simulink model "gm_sampleModel2077_2_sub"  (R2023a)
settings: Solver=VariableStepAuto  StartTime=0.0  StopTime=10.0  RelTol=1e-3
libraries: simulink x1, hdlsllib x1
settings Model: Creator=user1  LastModifiedBy=user1
settings OptimizationCC: BlockReduction=off  ConditionallyExecuteInputs=off
settings DebuggingCC: InheritedTsInSrcMsg=none

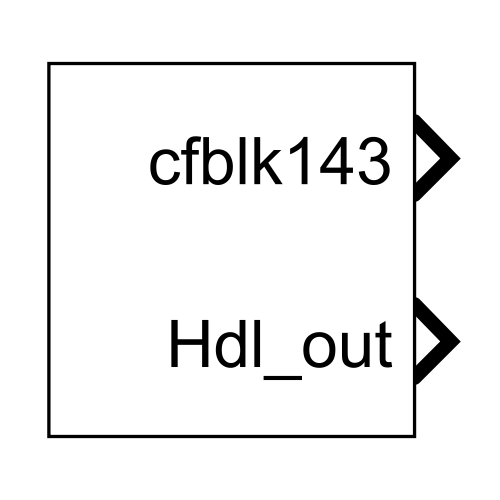
[thumbnail: Simulink's stored preview of the top-level diagram]
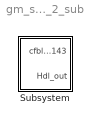
== system gm_sampleModel2077_2_sub ==
  Subsystem : Subsystem

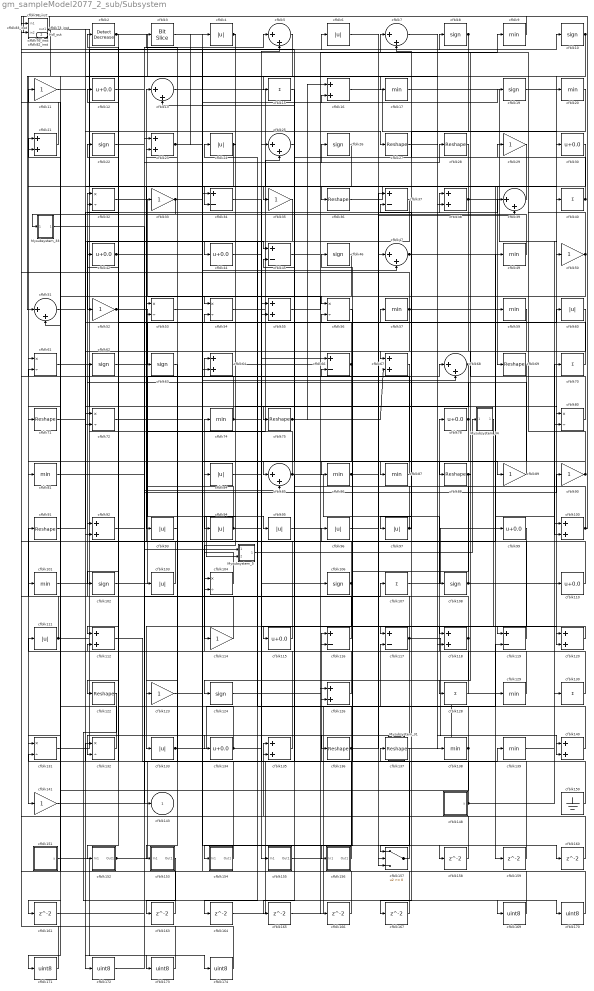
== system gm_sampleModel2077_2_sub/Subsystem ==
  Mysubsystem_31 : Subsystem
  Mysubsystem_33 : Subsystem
  Mysubsystem_34 : Subsystem
  Mysubsystem_5 : Subsystem
  cfblk{8,10,19,22,26,46,62..63,102,106,108,124} (12 alike) : Signum
  cfblk{16,21,23,38,55,64,67,92,100,112,118,120,126,135,140} (15 alike) : Sum  OutDataTypeStr=uint8
  cfblk{9,17,20,49,57,59,74,81,86..87,101,129,138..139} (14 alike) : MinMax  OutDataTypeStr=uint8
  cfblk{4,6,24,60,84,93..97,103,111,133} (13 alike) : Abs  OutDataTypeStr=uint8  SaturateOnIntegerOverflow=off
  cfblk{32,53..54,56,61,72,80,104,131..132} (10 alike) : Product  Inputs=*/  OutDataTypeStr=uint8  RndMeth=Zero  SaturateOnIntegerOverflow=on
  cfblk{15,40,70,107,128,130} (6 alike) : Sum  Inputs=+  OutDataTypeStr=uint8
  cfblk{11,29,33,35,50,52,89..90,114,123,141} (11 alike) : Gain  OutDataTypeStr=uint8
  cfblk{12,30,42,44,78,99,110,115,134} (9 alike) : Bias  Bias=0.0  SaturateOnIntegerOverflow=off
  cfblk{34,37,45,66,116..117,119} (7 alike) : Sum  Inputs=+-  OutDataTypeStr=uint8
  cfblk{27..28,36,69,71,75,88,91,122,136..137} (11 alike) : Reshape
  cfblk127_inst : Subsystem
  cfblk{5,7,13,25,39,47,51,68,85} (9 alike) : Sum  Inputs=|++  OutDataTypeStr=uint8
  cfblk148 : Subsystem  mask(Counter Free-Running){NumBits=double(16), tsamp=double(-1)}
      mask prompts: NumBits "Simulink:masks:NumberOfBits_MP"; tsamp "Simulink:masks:SampleTime_MP"
      mask help: Simulink:masks:CounterFreeRunning_MD
  cfblk14_inst : Subsystem
  cfblk150 : Ground
  cfblk151 : Subsystem  mask(Counter Limited){uplimit=double(7), tsamp=double(-1)}
      mask prompts: uplimit "Simulink:masks:UpperLimit_MP"; tsamp "Simulink:masks:SampleTime_MP"
      mask help: Simulink:masks:CounterLimited_MD
      mask init:
      | nbits = double(8);
      | tsamp = double(-1);
      | uplimit = double(7);
  cfblk152 : Subsystem
  cfblk153 : Subsystem
  cfblk154 : Subsystem
  cfblk155 : Subsystem
  cfblk156 : Subsystem
  cfblk157 : Switch  OutDataTypeStr=uint8  SaturateOnIntegerOverflow=off  InputSameDT=off
  cfblk{158..161,163..167} (9 alike) : Delay  SampleTime=1
  cfblk{169..174} (6 alike) : DataTypeConversion  OutDataTypeStr=uint8  SaturateOnIntegerOverflow=off  RndMeth=Floor
  cfblk18_inst : Subsystem
  cfblk2 : simulink/Logic and Bit Operations/Detect Decrease  vinit=0.0  OutDataTypeStr=uint8
      settings: LibrarySourceBlock=|
      | hdlsllib/Logic and Bit
      | Operations/Detect
      | Decrease
  cfblk3 : hdlsllib/Logic and Bit Operations/Bit Slice  lidx=7  ridx=0
  cfblk58_inst : Subsystem
  cfblk73_inst : Subsystem
  cfblk76_inst : Subsystem
  cfblk82_inst : Subsystem
  cfblk83_inst : Subsystem
  cfblk98_inst : Subsystem
  cfblk143 : Outport  OutDataTypeStr=uint8  SampleTime=1  VectorParamsAs1DForOutWhenUnconnected=off
  Hdl_out : Outport  Port=2  OutDataTypeStr=uint8
  wires:
  Mysubsystem_31/1(Out1) -> cfblk129/1
  Mysubsystem_33/1(Out1) -> Mysubsystem_5/1(In1)
  Mysubsystem_34/1(Out1) -> cfblk117/1
  Mysubsystem_5/1(Out1) -> Mysubsystem_34/1(In1)
  cfblk10/1 -> cfblk120/2, cfblk141/1
  cfblk100/1 -> cfblk14_inst/2(in2), cfblk61/2
  cfblk101/1 -> cfblk6/1
  cfblk102/1 -> cfblk68/1
  cfblk103/1 -> cfblk13/1
  cfblk104/1 -> cfblk74/1
  cfblk106/1 -> cfblk133/1, cfblk32/1
  cfblk107/1 -> cfblk99/1
  cfblk108/1 -> cfblk64/1, cfblk18_inst/1(in1), cfblk110/1
  cfblk11/1 -> cfblk72/1
  cfblk110/1 -> cfblk96/1
  cfblk111/1 -> cfblk91/1, cfblk25/2
  cfblk112/1 -> cfblk135/1
  cfblk114/1 -> cfblk92/1
  cfblk115/1 -> cfblk83_inst/1(in1)
  cfblk116/1 -> cfblk101/1
  cfblk117/1 -> cfblk82_inst/2(in2), cfblk140/2, cfblk127_inst/1(in1), cfblk132/2
  cfblk118/1 -> cfblk83_inst/2(in2), cfblk124/1
  cfblk119/1 -> cfblk11/1
  cfblk12/1 -> cfblk10/1
  cfblk120/1 -> cfblk115/1
  cfblk122/1 -> cfblk170/1
  cfblk123/1 -> cfblk8/1
  cfblk124/1 -> cfblk116/1
  cfblk126/1 -> cfblk84/1
  cfblk127_inst/1(out1) -> cfblk93/1, cfblk69/1, cfblk35/1
  cfblk128/1 -> cfblk78/1
  cfblk129/1 -> cfblk66/2
  cfblk13/1 -> cfblk159/1
  cfblk130/1 -> cfblk111/1
  cfblk131/1 -> cfblk49/1
  cfblk132/1 -> cfblk51/2
  cfblk133/1 -> cfblk119/2, cfblk53/1
  cfblk134/1 -> cfblk25/1, cfblk2/1
  cfblk135/1 -> cfblk24/1
  cfblk136/1 -> cfblk47/1, cfblk116/2, cfblk154/1(In1)
  cfblk137/1 -> cfblk157/1
  cfblk138/1 -> cfblk46/1, cfblk161/1
  cfblk139/1 -> cfblk70/1
  cfblk14_inst/1(out1) -> cfblk45/1, cfblk34/2
  cfblk140/1 -> cfblk54/2
  cfblk141/1 -> cfblk139/1
  cfblk148/1(y) -> cfblk56/2, cfblk132/1, cfblk130/1
  cfblk15/1 -> cfblk85/1
  cfblk150/1 -> cfblk112/2
  cfblk151/1(y) -> cfblk173/1
  cfblk152/1(Out1) -> cfblk55/2, cfblk5/2
  cfblk153/1(Out1) -> cfblk163/1
  cfblk154/1(Out1) -> cfblk23/2
  cfblk155/1(Out1) -> cfblk137/1
  cfblk156/1(Out1) -> cfblk21/1
  cfblk157/1 -> cfblk21/2
  cfblk158/1 -> cfblk58_inst/2(in2)
  cfblk159/1 -> cfblk45/2
  cfblk16/1 -> cfblk30/1
  cfblk160/1 -> cfblk135/2
  cfblk161/1 -> cfblk85/2
  cfblk163/1 -> cfblk23/1
  cfblk164/1 -> cfblk126/2
  cfblk165/1 -> cfblk117/2
  cfblk166/1 -> cfblk131/2
  cfblk167/1 -> cfblk127_inst/2(in2)
  cfblk169/1 -> cfblk34/1
  cfblk17/1 -> cfblk50/1
  cfblk170/1 -> cfblk76_inst/1(in1)
  cfblk171/1 -> cfblk76_inst/2(in2)
  cfblk172/1 -> cfblk107/1
  cfblk173/1 -> cfblk98_inst/1(in1)
  cfblk174/1 -> cfblk98_inst/2(in2)
  cfblk18_inst/1(out1) -> cfblk14_inst/1(in1)
  cfblk19/1 -> cfblk20/1
  cfblk2/1 -> cfblk122/1, cfblk118/2
  cfblk20/1 -> cfblk67/1
  cfblk21/1 -> cfblk82_inst/1(in1)
  cfblk22/1 -> cfblk5/1
  cfblk23/1 -> cfblk95/1, cfblk68/2, cfblk4/1
  cfblk24/1 -> cfblk92/2, cfblk114/1
  cfblk25/1 -> cfblk75/1
  cfblk26/1 -> cfblk71/1
  cfblk27/1 -> cfblk138/1
  cfblk28/1 -> cfblk54/1
  cfblk29/1 -> cfblk61/1
  cfblk3/1 -> cfblk88/1
  cfblk30/1 -> cfblk87/1
  cfblk32/1 -> cfblk166/1
  cfblk33/1 -> cfblk47/2, Mysubsystem_33/1(In1)
  cfblk34/1 -> cfblk155/1(In1)
  cfblk35/1 -> cfblk52/1
  cfblk36/1 -> cfblk40/1
  cfblk37/1 -> cfblk134/1
  cfblk38/1 -> cfblk64/2, cfblk100/1, cfblk33/1
  cfblk39/1 -> cfblk36/1
  cfblk4/1 -> cfblk44/1, cfblk104/2
  cfblk40/1 -> cfblk7/2, cfblk13/2
  cfblk42/1 -> cfblk26/1, cfblk16/2
  cfblk44/1 -> cfblk106/1
  cfblk45/1 -> cfblk9/1
  cfblk46/1 -> cfblk81/1
  cfblk47/1 -> cfblk97/1, cfblk100/2
  cfblk49/1 -> cfblk12/1
  cfblk5/1 -> cfblk131/1
  cfblk50/1 -> cfblk73_inst/2(in2), cfblk112/1
  cfblk51/1 -> cfblk80/1
  cfblk52/1 -> cfblk28/1, Mysubsystem_5/2(In2)
  cfblk53/1 -> cfblk38/1
  cfblk54/1 -> cfblk56/1
  cfblk55/1 -> cfblk19/1
  cfblk56/1 -> cfblk156/1(In1)
  cfblk57/1 -> cfblk18_inst/2(in2), cfblk72/2, cfblk59/1
  cfblk58_inst/1(out1) -> cfblk17/1
  cfblk59/1 -> cfblk128/1
  cfblk6/1 -> cfblk157/2
  cfblk60/1 -> cfblk152/1(In1)
  cfblk61/1 -> cfblk143/1
  cfblk62/1 -> cfblk55/1
  cfblk63/1 -> cfblk153/1(In1)
  cfblk64/1 -> cfblk80/2
  cfblk66/1 -> cfblk42/1, cfblk123/1
  cfblk67/1 -> cfblk94/1
  cfblk68/1 -> cfblk167/1, cfblk104/1
  cfblk69/1 -> cfblk102/1
  cfblk7/1 -> cfblk140/1
  cfblk70/1 -> cfblk32/2
  cfblk71/1 -> cfblk60/1
  cfblk72/1 -> cfblk158/1
  cfblk73_inst/1(out1) -> cfblk27/1
  cfblk74/1 -> cfblk22/1, cfblk89/1
  cfblk75/1 -> cfblk67/2, cfblk16/1
  cfblk76_inst/1(out1) -> cfblk169/1
  cfblk78/1 -> cfblk37/2, cfblk171/1, cfblk164/1
  cfblk8/1 -> cfblk38/2, cfblk15/1
  cfblk80/1 -> cfblk7/1
  cfblk81/1 -> cfblk103/1
  cfblk82_inst/1(out1) -> cfblk174/1
  cfblk83_inst/1(out1) -> cfblk51/1
  cfblk84/1 -> cfblk66/1
  cfblk85/1 -> cfblk108/1, cfblk53/2, cfblk165/1
  cfblk86/1 -> cfblk39/2, cfblk160/1
  cfblk87/1 -> cfblk73_inst/1(in1)
  cfblk88/1 -> cfblk136/1, cfblk118/1
  cfblk89/1 -> cfblk62/1
  cfblk9/1 -> cfblk58_inst/1(in1)
  cfblk90/1 -> cfblk29/1, cfblk86/1
  cfblk91/1 -> cfblk39/1
  cfblk92/1 -> cfblk90/1
  cfblk93/1 -> cfblk3/1
  cfblk94/1 -> cfblk63/1, cfblk120/1
  cfblk95/1 -> cfblk126/1
  cfblk96/1 -> cfblk157/3
  cfblk97/1 -> cfblk37/1, cfblk57/1
  cfblk98_inst/1(out1) -> cfblk172/1
  cfblk99/1 -> cfblk119/1

== system gm_sampleModel2077_2_sub/Subsystem/Mysubsystem_31 ==
  cfblk125_to_const : Constant  Value=double(1)  OutDataTypeStr=double  SampleTime=1
  Out1 : Outport  SampleTime=1
  wires:
  cfblk125_to_const/1 -> Out1/1

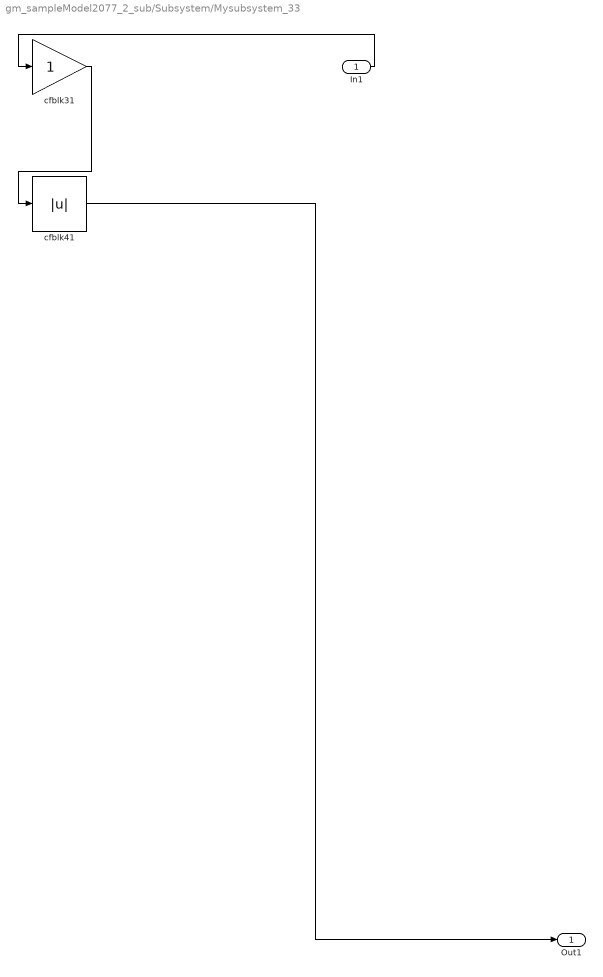
== system gm_sampleModel2077_2_sub/Subsystem/Mysubsystem_33 ==
  In1 : Inport  OutDataTypeStr=uint8  PortDimensions=1  SampleTime=1
  cfblk31 : Gain
  cfblk41 : Abs  SaturateOnIntegerOverflow=off
  Out1 : Outport  SampleTime=1
  wires:
  In1/1 -> cfblk31/1
  cfblk31/1 -> cfblk41/1
  cfblk41/1 -> Out1/1

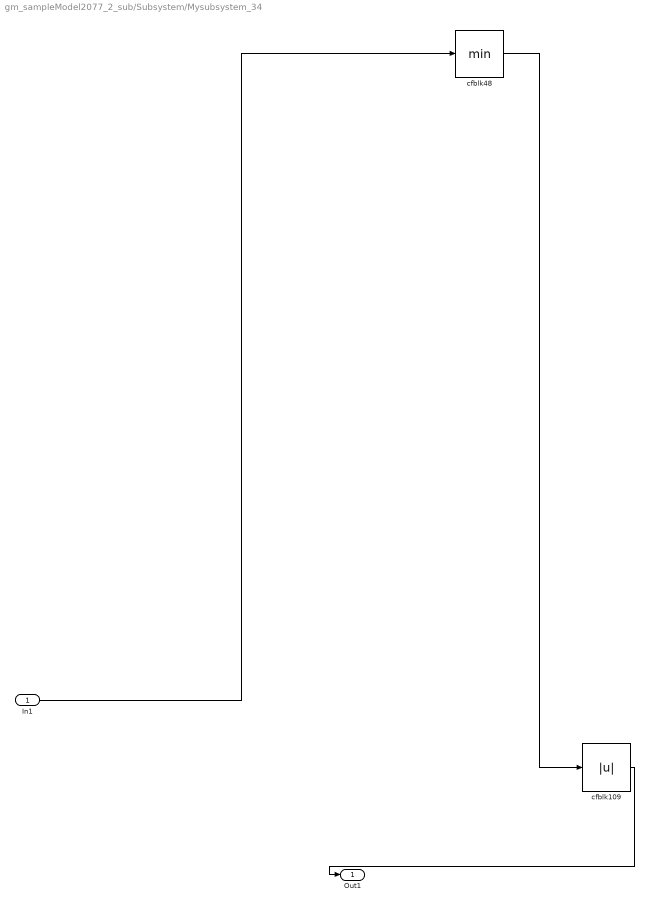
== system gm_sampleModel2077_2_sub/Subsystem/Mysubsystem_34 ==
  In1 : Inport  OutDataTypeStr=fixdt(0, 8, 7)  PortDimensions=1  SampleTime=1
  cfblk109 : Abs  SaturateOnIntegerOverflow=off
  cfblk48 : MinMax
  Out1 : Outport  SampleTime=1
  wires:
  In1/1 -> cfblk48/1
  cfblk109/1 -> Out1/1
  cfblk48/1 -> cfblk109/1

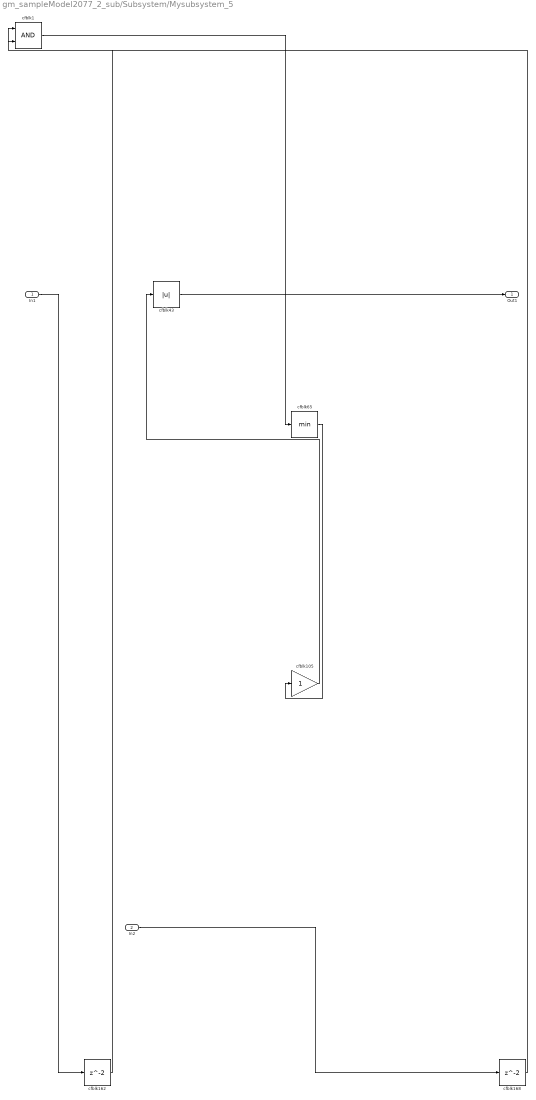
== system gm_sampleModel2077_2_sub/Subsystem/Mysubsystem_5 ==
  In1 : Inport  OutDataTypeStr=fixdt(0, 16, 7)  PortDimensions=1  SampleTime=1
  In2 : Inport  Port=2  OutDataTypeStr=uint8  PortDimensions=1  SampleTime=1
  cfblk1 : Logic  AllPortsSameDT=off  OutDataTypeStr=boolean
  cfblk105 : Gain
  cfblk162 : Delay  SampleTime=1
  cfblk168 : Delay  SampleTime=1
  cfblk43 : Abs  SaturateOnIntegerOverflow=off
  cfblk65 : MinMax
  Out1 : Outport  SampleTime=1
  wires:
  In1/1 -> cfblk162/1
  In2/1 -> cfblk168/1
  cfblk1/1 -> cfblk65/1
  cfblk105/1 -> cfblk43/1
  cfblk162/1 -> cfblk1/1
  cfblk168/1 -> cfblk1/2
  cfblk43/1 -> Out1/1
  cfblk65/1 -> cfblk105/1

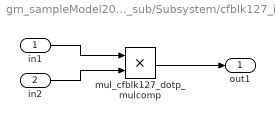
== system gm_sampleModel2077_2_sub/Subsystem/cfblk127_inst ==
  in1 : Inport  OutDataTypeStr=uint8  SampleTime=1
  in2 : Inport  Port=2  OutDataTypeStr=uint8  SampleTime=1
  mul_cfblk127_dotp_mulcomp : Product  Inputs=**  OutDataTypeStr=uint8  SampleTime=1
  out1 : Outport  OutDataTypeStr=uint8  SampleTime=1
  wires:
  in1/1 -> mul_cfblk127_dotp_mulcomp/1
  in2/1 -> mul_cfblk127_dotp_mulcomp/2
  mul_cfblk127_dotp_mulcomp/1 -> out1/1

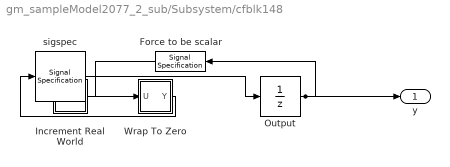
== system gm_sampleModel2077_2_sub/Subsystem/cfblk148 ==
  Force to be scalar : SignalSpecification  DisableCoverage=on  Dimensions=1
  Increment Real World : Subsystem  mask(Real World Value Increment){}
      mask help: Simulink:masks:RealWorldValueIncrement_MD
      mask Display: disp('V++')
  Output : UnitDelay  InitialCondition=0.0  SampleTime=tsamp  HasFrameUpgradeWarning=on
  Wrap To Zero : Subsystem  mask(Wrap To Zero){Threshold=double(65535)}
      mask prompts: Threshold "Simulink:masks:Threshold_MP"
      mask help: Simulink:masks:WrapToZero_MD
  sigspec : SignalSpecification  OutDataTypeStr=uint16  Dimensions=1
  y : Outport  SampleTime=1
  wires:
  Force to be scalar/1 -> Increment Real World/1(u)
  Increment Real World/1(y) -> Wrap To Zero/1(U)
  Output/1 -> Force to be scalar/1, y/1
  Wrap To Zero/1(Y) -> sigspec/1
  sigspec/1 -> Output/1

== system gm_sampleModel2077_2_sub/Subsystem/cfblk14_inst ==
  in1 : Inport  OutDataTypeStr=uint8  SampleTime=1
  in2 : Inport  Port=2  OutDataTypeStr=uint8  SampleTime=1
  mul_cfblk14_dotp_mulcomp : Product  Inputs=**  OutDataTypeStr=uint8  SampleTime=1
  out1 : Outport  OutDataTypeStr=uint8  SampleTime=1
  wires:
  in1/1 -> mul_cfblk14_dotp_mulcomp/1
  in2/1 -> mul_cfblk14_dotp_mulcomp/2
  mul_cfblk14_dotp_mulcomp/1 -> out1/1

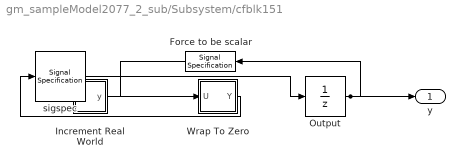
== system gm_sampleModel2077_2_sub/Subsystem/cfblk151 ==
  Force to be scalar : SignalSpecification  DisableCoverage=on  Dimensions=1
  Increment Real World : Subsystem  mask(Real World Value Increment){}
      mask help: Simulink:masks:RealWorldValueIncrement_MD
      mask Display: disp('V++')
  Output : UnitDelay  InitialCondition=0.0  SampleTime=tsamp  HasFrameUpgradeWarning=on
  Wrap To Zero : Subsystem  mask(Wrap To Zero){Threshold=double(7)}
      mask prompts: Threshold "Simulink:masks:Threshold_MP"
      mask help: Simulink:masks:WrapToZero_MD
  sigspec : SignalSpecification  OutDataTypeStr=uint8  Dimensions=1
  y : Outport  SampleTime=1
  wires:
  Force to be scalar/1 -> Increment Real World/1(u)
  Increment Real World/1(y) -> Wrap To Zero/1(U)
  Output/1 -> Force to be scalar/1, y/1
  Wrap To Zero/1(Y) -> sigspec/1
  sigspec/1 -> Output/1

== system gm_sampleModel2077_2_sub/Subsystem/cfblk152 ==
  In1 : Inport  OutDataTypeStr=uint8  PortDimensions=1  SampleTime=1
  Out1 : Outport  SampleTime=1
  wires:
  In1/1 -> Out1/1

== system gm_sampleModel2077_2_sub/Subsystem/cfblk153 ==
  In1 : Inport  OutDataTypeStr=uint8  PortDimensions=1  SampleTime=1
  Out1 : Outport  SampleTime=1
  wires:
  In1/1 -> Out1/1

== system gm_sampleModel2077_2_sub/Subsystem/cfblk154 ==
  In1 : Inport  OutDataTypeStr=uint8  PortDimensions=1  SampleTime=1
  Out1 : Outport  SampleTime=1
  wires:
  In1/1 -> Out1/1

== system gm_sampleModel2077_2_sub/Subsystem/cfblk155 ==
  In1 : Inport  OutDataTypeStr=uint8  PortDimensions=1  SampleTime=1
  Out1 : Outport  SampleTime=1
  wires:
  In1/1 -> Out1/1

== system gm_sampleModel2077_2_sub/Subsystem/cfblk156 ==
  In1 : Inport  OutDataTypeStr=uint8  PortDimensions=1  SampleTime=1
  Out1 : Outport  SampleTime=1
  wires:
  In1/1 -> Out1/1

== system gm_sampleModel2077_2_sub/Subsystem/cfblk18_inst ==
  in1 : Inport  OutDataTypeStr=uint8  SampleTime=1
  in2 : Inport  Port=2  OutDataTypeStr=uint8  SampleTime=1
  mul_cfblk18_dotp_mulcomp : Product  Inputs=**  OutDataTypeStr=uint8  SampleTime=1
  out1 : Outport  OutDataTypeStr=uint8  SampleTime=1
  wires:
  in1/1 -> mul_cfblk18_dotp_mulcomp/1
  in2/1 -> mul_cfblk18_dotp_mulcomp/2
  mul_cfblk18_dotp_mulcomp/1 -> out1/1

== system gm_sampleModel2077_2_sub/Subsystem/cfblk58_inst ==
  in1 : Inport  OutDataTypeStr=uint8  SampleTime=1
  in2 : Inport  Port=2  OutDataTypeStr=uint8  SampleTime=1
  mul_cfblk58_dotp_mulcomp : Product  Inputs=**  OutDataTypeStr=uint8  SampleTime=1
  out1 : Outport  OutDataTypeStr=uint8  SampleTime=1
  wires:
  in1/1 -> mul_cfblk58_dotp_mulcomp/1
  in2/1 -> mul_cfblk58_dotp_mulcomp/2
  mul_cfblk58_dotp_mulcomp/1 -> out1/1

== system gm_sampleModel2077_2_sub/Subsystem/cfblk73_inst ==
  in1 : Inport  OutDataTypeStr=uint8  SampleTime=1
  in2 : Inport  Port=2  OutDataTypeStr=uint8  SampleTime=1
  mul_cfblk73_dotp_mulcomp : Product  Inputs=**  OutDataTypeStr=uint8  SampleTime=1
  out1 : Outport  OutDataTypeStr=uint8  SampleTime=1
  wires:
  in1/1 -> mul_cfblk73_dotp_mulcomp/1
  in2/1 -> mul_cfblk73_dotp_mulcomp/2
  mul_cfblk73_dotp_mulcomp/1 -> out1/1

== system gm_sampleModel2077_2_sub/Subsystem/cfblk76_inst ==
  in1 : Inport  OutDataTypeStr=uint8  SampleTime=1
  in2 : Inport  Port=2  OutDataTypeStr=uint8  SampleTime=1
  mul_cfblk76_dotp_mulcomp : Product  Inputs=**  OutDataTypeStr=uint8  SampleTime=1
  out1 : Outport  OutDataTypeStr=uint8  SampleTime=1
  wires:
  in1/1 -> mul_cfblk76_dotp_mulcomp/1
  in2/1 -> mul_cfblk76_dotp_mulcomp/2
  mul_cfblk76_dotp_mulcomp/1 -> out1/1

== system gm_sampleModel2077_2_sub/Subsystem/cfblk82_inst ==
  in1 : Inport  OutDataTypeStr=uint8  SampleTime=1
  in2 : Inport  Port=2  OutDataTypeStr=uint8  SampleTime=1
  mul_cfblk82_dotp_mulcomp : Product  Inputs=**  OutDataTypeStr=uint8  SampleTime=1
  out1 : Outport  OutDataTypeStr=uint8  SampleTime=1
  wires:
  in1/1 -> mul_cfblk82_dotp_mulcomp/1
  in2/1 -> mul_cfblk82_dotp_mulcomp/2
  mul_cfblk82_dotp_mulcomp/1 -> out1/1

== system gm_sampleModel2077_2_sub/Subsystem/cfblk83_inst ==
  in1 : Inport  OutDataTypeStr=uint8  SampleTime=1
  in2 : Inport  Port=2  OutDataTypeStr=uint8  SampleTime=1
  mul_cfblk83_dotp_mulcomp : Product  Inputs=**  OutDataTypeStr=uint8  SampleTime=1
  out1 : Outport  OutDataTypeStr=uint8  SampleTime=1
  wires:
  in1/1 -> mul_cfblk83_dotp_mulcomp/1
  in2/1 -> mul_cfblk83_dotp_mulcomp/2
  mul_cfblk83_dotp_mulcomp/1 -> out1/1

== system gm_sampleModel2077_2_sub/Subsystem/cfblk98_inst ==
  in1 : Inport  OutDataTypeStr=uint8  SampleTime=1
  in2 : Inport  Port=2  OutDataTypeStr=uint8  SampleTime=1
  mul_cfblk98_dotp_mulcomp : Product  Inputs=**  OutDataTypeStr=uint8  SampleTime=1
  out1 : Outport  OutDataTypeStr=uint8  SampleTime=1
  wires:
  in1/1 -> mul_cfblk98_dotp_mulcomp/1
  in2/1 -> mul_cfblk98_dotp_mulcomp/2
  mul_cfblk98_dotp_mulcomp/1 -> out1/1

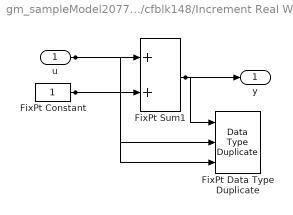
== system gm_sampleModel2077_2_sub/Subsystem/cfblk148/Increment Real World ==
  u : Inport  OutDataTypeStr=uint16  SampleTime=1
  FixPt Constant : Constant  DisableCoverage=on  OutDataTypeStr=Inherit: Inherit via back propagation  SampleTime=-1
  FixPt Data Type Duplicate : DataTypeDuplicate  DisableCoverage=on  NumInputPorts=3
  FixPt Sum1 : Sum  InputSameDT=on  OutDataTypeStr=Inherit: Inherit via back propagation  LockScale=on
  y : Outport  SampleTime=1
  wires:
  u/1 -> FixPt Sum1/1, FixPt Data Type Duplicate/2
  FixPt Constant/1 -> FixPt Sum1/2, FixPt Data Type Duplicate/3
  FixPt Sum1/1 -> FixPt Data Type Duplicate/1, y/1

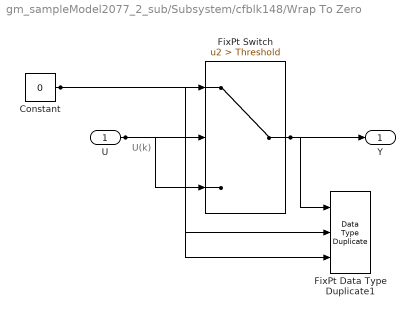
== system gm_sampleModel2077_2_sub/Subsystem/cfblk148/Wrap To Zero ==
  note: U(k)
  U : Inport  OutDataTypeStr=uint16  SampleTime=1
  Constant : Constant  DisableCoverage=on  Value=0  OutDataTypeStr=Inherit: Inherit via back propagation  SampleTime=-1
  FixPt Data Type Duplicate1 : DataTypeDuplicate  DisableCoverage=on  NumInputPorts=3
  FixPt Switch : Switch  Criteria=u2 > Threshold  Threshold=Threshold  OutDataTypeStr=Inherit: Inherit via back propagation  ZeroCross=off  SaturateOnIntegerOverflow=off  InputSameDT=off
  Y : Outport  SampleTime=1
  wires:
  U/1 -> FixPt Switch/3, FixPt Switch/2, FixPt Data Type Duplicate1/2
  Constant/1 -> FixPt Switch/1, FixPt Data Type Duplicate1/3
  FixPt Switch/1 -> FixPt Data Type Duplicate1/1, Y/1

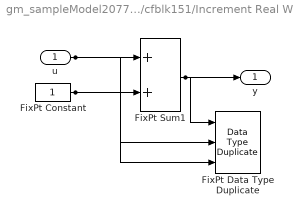
== system gm_sampleModel2077_2_sub/Subsystem/cfblk151/Increment Real World ==
  u : Inport  OutDataTypeStr=uint8  SampleTime=1
  FixPt Constant : Constant  DisableCoverage=on  OutDataTypeStr=Inherit: Inherit via back propagation  SampleTime=-1
  FixPt Data Type Duplicate : DataTypeDuplicate  DisableCoverage=on  NumInputPorts=3
  FixPt Sum1 : Sum  InputSameDT=on  OutDataTypeStr=Inherit: Inherit via back propagation  LockScale=on
  y : Outport  SampleTime=1
  wires:
  u/1 -> FixPt Sum1/1, FixPt Data Type Duplicate/2
  FixPt Constant/1 -> FixPt Sum1/2, FixPt Data Type Duplicate/3
  FixPt Sum1/1 -> FixPt Data Type Duplicate/1, y/1

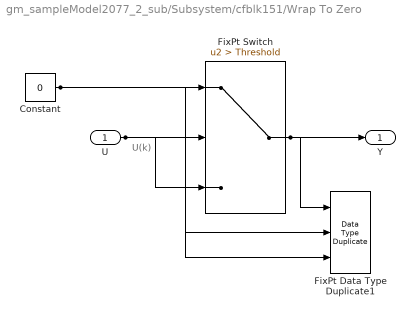
== system gm_sampleModel2077_2_sub/Subsystem/cfblk151/Wrap To Zero ==
  note: U(k)
  U : Inport  OutDataTypeStr=uint8  SampleTime=1
  Constant : Constant  DisableCoverage=on  Value=0  OutDataTypeStr=Inherit: Inherit via back propagation  SampleTime=-1
  FixPt Data Type Duplicate1 : DataTypeDuplicate  DisableCoverage=on  NumInputPorts=3
  FixPt Switch : Switch  Criteria=u2 > Threshold  Threshold=Threshold  OutDataTypeStr=Inherit: Inherit via back propagation  ZeroCross=off  SaturateOnIntegerOverflow=off  InputSameDT=off
  Y : Outport  SampleTime=1
  wires:
  U/1 -> FixPt Switch/3, FixPt Switch/2, FixPt Data Type Duplicate1/2
  Constant/1 -> FixPt Switch/1, FixPt Data Type Duplicate1/3
  FixPt Switch/1 -> FixPt Data Type Duplicate1/1, Y/1
